simulink model "serratura_riccio"  (Simulink 10.0)
settings: Solver=FixedStepDiscrete  StartTime=0.0  StopTime=5  FixedStep=1  RelTol=1e-3  AbsTol=1e-6  EnableMultiTasking=on
settings Model: Creator=prof. G. Celentano  LastModifiedBy=giuseppericcio  ExtModeTrigMode=oneshot  ExtModeArmWhenConnect=off
settings SolverCC: AutoScaleAbsTol=off
settings DataIOCC: SignalLoggingSaveFormat=ModelDataLogs  SignalLoggingName=sigsOut
settings OptimizationCC: BooleanDataType=off  ExpressionDepthLimit=2147483647  InitFltsAndDblsToZero=on
settings DebuggingCC: SaveWithParameterizedLinksMsg=none  SignalResolutionControl=TryResolveAllWithWarning  MultiTaskDSMMsg=warning  MultiTaskCondExecSysMsg=none  FcnCallInpInsideContextMsg=warning  StateNameClashWarn=warning
settings HardwareCC: TargetUnknown=on
settings GRTTargetCC: TargetFcnLib=ansi_tfl_tmw.mat

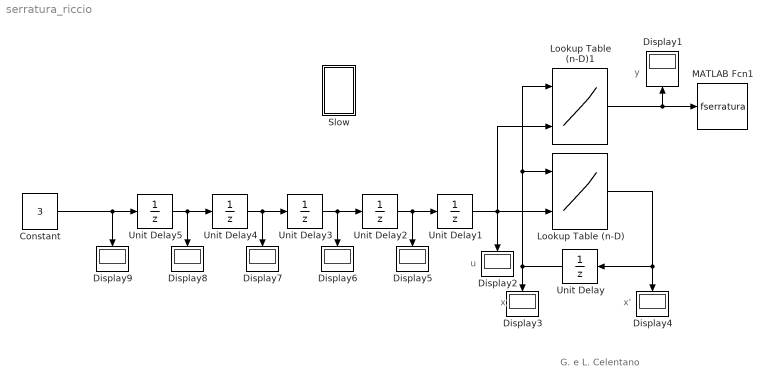
== system serratura_riccio ==
  note: G. e L. Celentano
  note: u
  note: x
  note: y
  note: x'
  Constant : Constant  Value=3
  Display{1..9} (9 alike) : Display
  Lookup Table (n-D) : Lookup_n-D  BreakpointsForDimension1=[1,2,3,4,5,6]  BreakpointsForDimension2=[1,2,3,4]  IndexSearchMethod=Linear search  Table=reshape([1,1,4,5,1,1,1,3,1,1,6,1,1,1,1,1,1,1,2,2,2,2,2,2],6,4)  InputSameDT=on
  Lookup Table (n-D)1 : Lookup_n-D  BreakpointsForDimension1=[1,2,3,4,5,6]  BreakpointsForDimension2=[1,2,3,4]  IndexSearchMethod=Linear search  Table=reshape([1,1,1,1,1,1,1,1,1,1,1,1,1,1,1,1,1,2,1,1,1,1,1,1],6,4)  InputSameDT=on
  MATLAB Fcn1 : MATLABFcn  MATLABFcn=fserratura  OutputDimensions=0
  Slow : Subsystem
      mask Display: plot([0 1],[0 1])
  Unit Delay : UnitDelay  InitialCondition=1
  Unit Delay1 : UnitDelay  InitialCondition=4
  Unit Delay2 : UnitDelay  InitialCondition=2
  Unit Delay3 : UnitDelay  InitialCondition=1
  Unit Delay4 : UnitDelay  InitialCondition=1
  Unit Delay5 : UnitDelay  InitialCondition=2
  wires:
  Lookup Table (n-D)/1 -> Unit Delay/1, Display4/1
  Unit Delay1/1 -> Display2/1, Lookup Table (n-D)/2, Lookup Table (n-D)1/2
  Lookup Table (n-D)1/1 -> Display1/1, MATLAB Fcn1/1
  Unit Delay2/1 -> Unit Delay1/1, Display5/1
  Unit Delay3/1 -> Unit Delay2/1, Display6/1
  Unit Delay4/1 -> Display7/1, Unit Delay3/1
  Unit Delay/1 -> Lookup Table (n-D)1/1, Lookup Table (n-D)/1, Display3/1
  Unit Delay5/1 -> Display8/1, Unit Delay4/1
  Constant/1 -> Display9/1, Unit Delay5/1

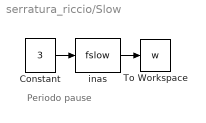
== system serratura_riccio/Slow ==
  note: Periodo
      | pause
  Constant : Constant  Value=3
  To Workspace : ToWorkspace  VariableName=w  SampleTime=-1
  inas : MATLABFcn  MATLABFcn=fslow
  wires:
  Constant/1 -> inas/1
  inas/1 -> To Workspace/1
